simulink model "CollectionData_Template_2019b"  (R2019b)
settings: Solver=ode1  StartTime=0.0  StopTime=60  FixedStep=0.002  RelTol=1e-3  EnableMultiTasking=on
PostLoadFcn:
  | qc_set_target_type(getConfigSet(bdroot, 'QUARC Default Target Configuration'));
undefined symbols (not defined in the file or in its folder): HIL, K_eta, K_x, L, qc_get_step_size, sysestc
libraries: simulink_extras x6, quarc_library x6, cstblocks x1
settings Model: SimulationMode=external  ExtModeTrigDuration=5000  Creator=CFulford  LastModifiedBy=Student
settings SolverCC: PositivePriorityOrder=on
settings DataIOCC: LimitDataPoints=on  SaveFormat=Array  SignalLoggingSaveFormat=ModelDataLogs  ReturnWorkspaceOutputs=off
settings OptimizationCC: ExpressionDepthLimit=2147483647  InitFltsAndDblsToZero=on  LifeSpan=inf
settings DebuggingCC: SaveWithParameterizedLinksMsg=none  UnderspecifiedInitializationDetection=Classic  MergeDetectMultiDrivingBlocksExec=none  SolverPrmCheckMsg=warning  MultiTaskDSMMsg=warning  MultiTaskCondExecSysMsg=none  FcnCallInpInsideContextMsg=warning  StateNameClashWarn=warning  SFUnexpectedBacktrackingDiag=warning  SFNoUnconditionalDefaultTransitionDiag=warning  SFExecutionAtInitializationDiag=none  ArithmeticOperatorsInVariantConditions=warning
settings HardwareCC: ProdBitPerPointer=32  ProdBitPerSizeT=32  ProdBitPerPtrDiffT=32  ProdLargestAtomicFloat=None  ProdIntDivRoundTo=Undefined  ProdEndianess=Unspecified  ProdWordSize=32  ProdHWDeviceType=32-bit Generic
settings ModelReferenceCC: PropagateSignalLabelsOutOfModel=off
settings SFSimCC: SimUseLocalCustomCode=off  CustomCodeUndefinedFunction=UseInterfaceOnly
settings RTWCC: Description=QUARC Win64 Target  SystemTargetFile=quarc_win64.tlc  TemplateMakefile=quarc_default_tmf  RTWUseLocalCustomCode=off
settings CodeAppCC: StateflowObjectComments=on
settings STFCustomTargetCC: TargetPreCompLibLocation=C:\PROGRA~3\QUARC\lib\2019b\win64\release  ConcurrentExecutionCompliant=on  CombineOutputUpdateFcns=on  CPPClassGenCompliant=on  SystemTargetFile=quarc_win64.tlc
settings GRTTargetCC: TargetPreCompLibLocation=C:\PROGRA~3\QUARC\lib\2019b\win64\release  TargetLangStandard=C89/C90 (ANSI)  ParMdlRefBuildCompliant=off  CompOptLevelCompliant=off  MatFileLogging=off  UseToolchainInfoCompliant=off  ExtMode=on  ExtModeMexFile=quarc_comm
settings ConfigComp: CovMetricSettings=dw  CovSaveCumulativeToWorkspaceVar=on  CovSaveSingleToWorkspaceVar=on  CovExternalEMLEnable=off  CovSFcnEnable=off

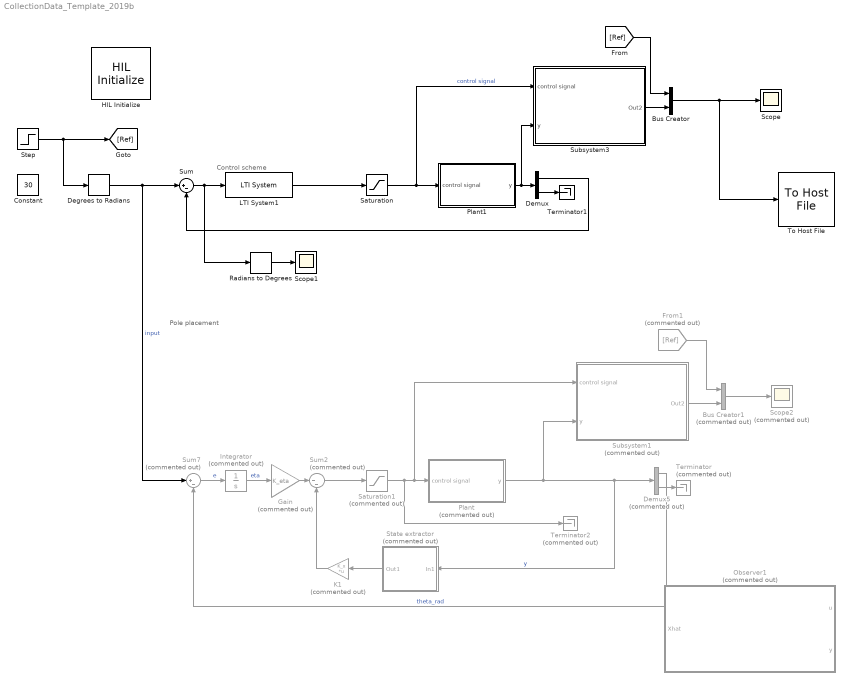
== system CollectionData_Template_2019b ==
  note: Control scheme
  note: Pole placement
  Bus Creator : BusCreator  Inputs=2
  Bus Creator1 : BusCreator  Commented=on  Inputs=2
  Constant : Constant  Value=30
  Degrees to Radians : simulink_extras/Transformations/Degrees to Radians
  Demux : Demux  Outputs=2
  Demux5 : Demux  Commented=on  Outputs=2
  From1 : From  Commented=on  GotoTag=Ref
  Gain : Gain  Commented=on  Gain=K_eta
  HIL Initialize : quarc_library/Data Acquisition/Generic/Configuration/HIL Initialize  Priority=-99  object_name=HIL-1  board_type=q2_usb  board_number=0  board_options=d0=digital;d1=digital;led=auto;update_rate=normal;decimation=1  exclusive=off  active=off  hardware_clocks=[0]  clock_modes=[]  initial_clock_frequencies=[]  set_clock_params_at_start=off  set_clock_params_at_switch_in=off  set_clock_frequencies_at_start=off  set_clock_frequencies_at_switch_in=off  analog_input_channels=[0:1]  analog_input_configurations=[]  analog_input_maximums=10  analog_input_minimums=-10  set_analog_input_params_at_start=on  set_analog_input_params_at_switch_in=off  analog_output_channels=[0:1]  analog_output_maximums=10  analog_output_minimums=-10  initial_analog_outputs=[0]  final_analog_outputs=[0]  watchdog_analog_outputs=0  set_analog_output_params_at_start=on  set_analog_output_params_at_switch_in=off  set_analog_outputs_at_start=on  set_analog_outputs_at_switch_in=off  set_analog_outputs_at_terminate=on  set_analog_outputs_at_switch_out=off  set_analog_outputs_on_watchdog=off  digital_input_channels=[]  digital_output_channels=[]  digital_output_configuration=[]  initial_digital_outputs=[1]  final_digital_outputs=[1]  watchdog_digital_outputs=[1]  set_digital_output_params_at_start=off  set_digital_output_params_at_switch_in=off  set_digital_outputs_at_start=on  set_digital_outputs_at_switch_in=off  set_digital_outputs_at_terminate=on  set_digital_outputs_at_switch_out=off  set_digital_outputs_on_watchdog=off  encoder_channels=[0:1]  quadrature=[4]  encoder_filter_frequency=[]  initial_encoder_counts=[0]  set_encoder_params_at_start=on  set_encoder_params_at_switch_in=off  set_encoder_counts_at_start=on  set_encoder_counts_at_switch_in=off  pwm_channels=[]  pwm_modes=[0]  pwm_frequency=1/0.020  pwm_configuration=[]  pwm_alignment=[]  pwm_polarity=[]  pwm_leading_deadband=[]  pwm_trailing_deadband=[]  initial_pwm_outputs=[0]  final_pwm_outputs=[0]  watchdog_pwm_outputs=[0]  set_pwm_params_at_start=on  set_pwm_params_at_switch_in=off  set_pwm_outputs_at_start=on  set_pwm_outputs_at_switch_in=off  set_pwm_outputs_at_terminate=on  set_pwm_outputs_at_switch_out=off  set_pwm_outputs_on_watchdog=off  other_output_channels=[]  initial_other_outputs=[]  final_other_outputs=[]  watchdog_other_outputs=[]  set_other_outputs_at_start=off  set_other_outputs_at_switch_in=off  set_other_outputs_at_terminate=off  set_other_outputs_at_switch_out=off  set_other_outputs_on_watchdog=off
  Integrator : Integrator  Commented=on
  K1 : Gain  Commented=on  Gain=K_x  Multiplication=Matrix(K*u)
  LTI System1 : cstblocks/LTI System  sys=syscomp_JC  IC=[]
  Observer1 : Subsystem  Commented=on
  Plant : Subsystem  Commented=on
  Plant1 : Subsystem
  Radians to Degrees : simulink_extras/Transformations/Radians to Degrees
  Saturation : Saturate  UpperLimit=10  LowerLimit=-10
  Saturation1 : Saturate  Commented=on  UpperLimit=4.5  LowerLimit=-4.5
  Scope : Scope
  Scope1 : Scope
  Scope2 : Scope  Commented=on
  State extractor : Subsystem  Commented=on
  Step : Step  After=30  SampleTime=0
  Subsystem1 : Subsystem  Commented=on
  Subsystem3 : Subsystem
  Sum : Sum  Inputs=|+-
  Sum2 : Sum  Commented=on  Inputs=|--
  Sum7 : Sum  Commented=on  Inputs=|+-
  Terminator : Terminator  Commented=on
  Terminator1 : Terminator
  Terminator2 : Terminator  Commented=on
  To Host File : quarc_library/Sinks/To Host/To Host File  file_name=JC_compensator.mat  variable_name=data  decimation=1  sample_time=-1  file_format=MAT-file v.4  options=No header or footer  append=off  final_file_name=JC_compensator.mat  bitrate=2000000
  wires:
  Sum/1 -> Radians to Degrees/1, LTI System1/1
  LTI System1/1 -> Saturation/1
  Saturation/1 -> Plant1/1(control signal), Subsystem3/1(control signal)  "control signal"
  Demux/1 -> Sum/2
  Subsystem3/1(Out2) -> Bus Creator/2
  [Ref] -> Bus Creator/1
  Bus Creator/1 -> To Host File/1, Scope/1
  Radians to Degrees/1 -> Scope1/1
  K1/1 -> Sum2/2
  Sum2/1 -> Saturation1/1
  Plant/1(y) -> Subsystem1/2(y), State extractor/1(In1), Demux5/1  "y"
  Degrees to Radians/1 -> Sum7/1, Sum/1  "input"
  Saturation1/1 -> Terminator2/1, Subsystem1/1(control signal), Plant/1(control signal)
  Integrator/1 -> Gain/1  "eta"
  Sum7/1 -> Integrator/1  "e"
  Gain/1 -> Sum2/1
  Demux5/1 -> Sum7/2  "theta_rad"
  Subsystem1/1(Out2) -> Bus Creator1/2
  Bus Creator1/1 -> Scope2/1
  Demux5/2 -> Terminator/1
  From1/1 -> Bus Creator1/1
  Plant1/1(y) -> Subsystem3/2(y), Demux/1
  Demux/2 -> Terminator1/1
  State extractor/1(Out1) -> K1/1
  Step/1 -> Degrees to Radians/1, [Ref]

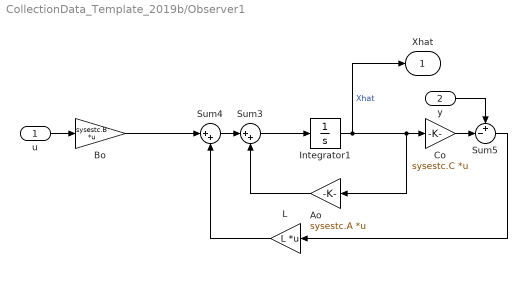
== system CollectionData_Template_2019b/Observer1 ==
  u : Inport
  y : Inport  Port=2
  Ao : Gain  Gain=sysestc.A  Multiplication=Matrix(K*u)
  Bo : Gain  Gain=sysestc.B  Multiplication=Matrix(K*u)
  Co : Gain  Gain=sysestc.C  Multiplication=Matrix(K*u)
  Integrator1 : Integrator
  L : Gain  Gain=L  Multiplication=Matrix(K*u)
  Sum3 : Sum  Inputs=|++
  Sum4 : Sum  Inputs=|++
  Sum5 : Sum  Inputs=+-|
  Xhat : Outport
  wires:
  Sum5/1 -> L/1
  Sum4/1 -> Sum3/1
  u/1 -> Bo/1
  Sum3/1 -> Integrator1/1
  Integrator1/1 -> Xhat/1, Ao/1, Co/1  "Xhat"
  Ao/1 -> Sum3/2
  L/1 -> Sum4/2
  Co/1 -> Sum5/2
  Bo/1 -> Sum4/1
  y/1 -> Sum5/1

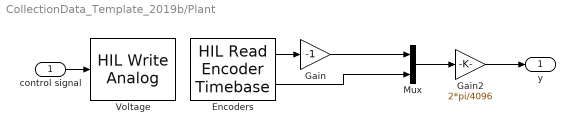
== system CollectionData_Template_2019b/Plant ==
  control signal : Inport
  Encoders : quarc_library/Data Acquisition/Generic/Timebases/HIL Read Encoder Timebase  object_name=HIL-1  clock=0  channels=[0:1]  samples_in_buffer=max(ceil(1/qc_get_step_size), 1)  active=on  vector_output=off  data_type_mode=Inherit via back propagation  data_type=double
  Gain : Gain  Gain=-1
  Gain2 : Gain  Gain=2*pi/4096
  Mux : Mux  Inputs=2
  Voltage : quarc_library/Data Acquisition/Generic/Immediate I//O/HIL Write Analog  object_name=HIL-1  channels=0  sample_time=-1  active=off  vector_input=off
  y : Outport
  wires:
  Encoders/1 -> Gain/1
  Encoders/2 -> Mux/2
  control signal/1 -> Voltage/1
  Mux/1 -> Gain2/1
  Gain/1 -> Mux/1
  Gain2/1 -> y/1

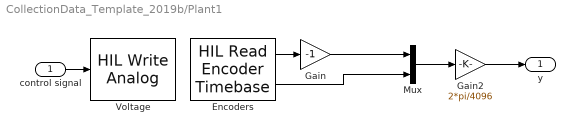
== system CollectionData_Template_2019b/Plant1 ==
  control signal : Inport
  Encoders : quarc_library/Data Acquisition/Generic/Timebases/HIL Read Encoder Timebase  object_name=HIL-1  clock=0  channels=[0:1]  samples_in_buffer=max(ceil(1/qc_get_step_size), 1)  active=on  vector_output=off  data_type_mode=Inherit via back propagation  data_type=double
  Gain : Gain  Gain=-1
  Gain2 : Gain  Gain=2*pi/4096
  Mux : Mux  Inputs=2
  Voltage : quarc_library/Data Acquisition/Generic/Immediate I//O/HIL Write Analog  object_name=HIL-1  channels=0  sample_time=-1  active=off  vector_input=off
  y : Outport
  wires:
  Encoders/1 -> Gain/1
  Encoders/2 -> Mux/2
  control signal/1 -> Voltage/1
  Mux/1 -> Gain2/1
  Gain/1 -> Mux/1
  Gain2/1 -> y/1

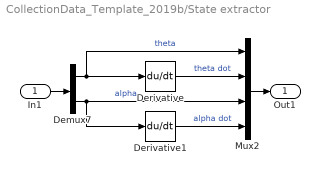
== system CollectionData_Template_2019b/State extractor ==
  In1 : Inport
  Demux7 : Demux  Outputs=2
  Derivative : Derivative
  Derivative1 : Derivative
  Mux2 : Mux
  Out1 : Outport
  wires:
  In1/1 -> Demux7/1
  Derivative1/1 -> Mux2/4  "alpha dot"
  Derivative/1 -> Mux2/2  "theta dot"
  Demux7/1 -> Mux2/1, Derivative/1  "theta"
  Demux7/2 -> Derivative1/1, Mux2/3  "alpha"
  Mux2/1 -> Out1/1

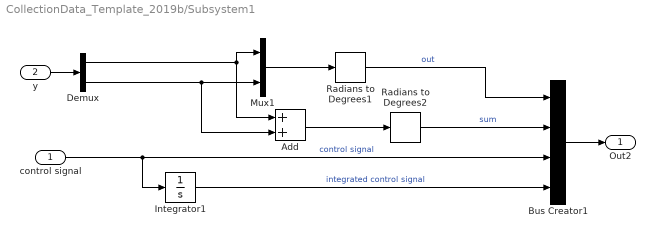
== system CollectionData_Template_2019b/Subsystem1 ==
  control signal : Inport
  y : Inport  Port=2
  Add : Sum
  Bus Creator1 : BusCreator  Inputs=4
  Demux : Demux  Outputs=2
  Integrator1 : Integrator
  Mux1 : Mux  Inputs=2
  Radians to Degrees1 : simulink_extras/Transformations/Radians to Degrees
  Radians to Degrees2 : simulink_extras/Transformations/Radians to Degrees
  Out2 : Outport
  wires:
  Mux1/1 -> Radians to Degrees1/1
  Radians to Degrees2/1 -> Bus Creator1/2  "sum"
  Bus Creator1/1 -> Out2/1
  Radians to Degrees1/1 -> Bus Creator1/1  "out"
  Integrator1/1 -> Bus Creator1/4  "integrated control signal"
  Demux/1 -> Mux1/1, Add/1
  Add/1 -> Radians to Degrees2/1
  control signal/1 -> Integrator1/1, Bus Creator1/3  "control signal"
  y/1 -> Demux/1
  Demux/2 -> Add/2, Mux1/2

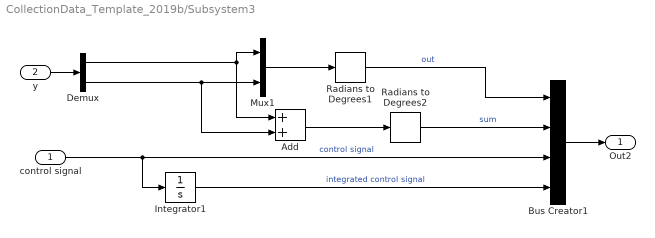
== system CollectionData_Template_2019b/Subsystem3 ==
  control signal : Inport
  y : Inport  Port=2
  Add : Sum
  Bus Creator1 : BusCreator  Inputs=4
  Demux : Demux  Outputs=2
  Integrator1 : Integrator
  Mux1 : Mux  Inputs=2
  Radians to Degrees1 : simulink_extras/Transformations/Radians to Degrees
  Radians to Degrees2 : simulink_extras/Transformations/Radians to Degrees
  Out2 : Outport
  wires:
  Mux1/1 -> Radians to Degrees1/1
  Radians to Degrees2/1 -> Bus Creator1/2  "sum"
  Bus Creator1/1 -> Out2/1
  Radians to Degrees1/1 -> Bus Creator1/1  "out"
  Integrator1/1 -> Bus Creator1/4  "integrated control signal"
  Demux/1 -> Mux1/1, Add/1
  Add/1 -> Radians to Degrees2/1
  control signal/1 -> Integrator1/1, Bus Creator1/3  "control signal"
  y/1 -> Demux/1
  Demux/2 -> Add/2, Mux1/2
